simulink model "signal_processing_simulink_hw1"  (R2017b)
settings: Solver=FixedStepAuto  StartTime=0.0  StopTime=2  FixedStep=0.01  RelTol=1e-3
values from neighbouring files (symbols this model uses):
  f = fl(k)    [signal_processing_hw1.m]
  M2 = 5    [signal_processing_hw1.m]
libraries: commchan3 x1
settings Model: Creator=nlztrk  LastModifiedBy=anilo
settings CodeAppCC: StateflowObjectComments=on

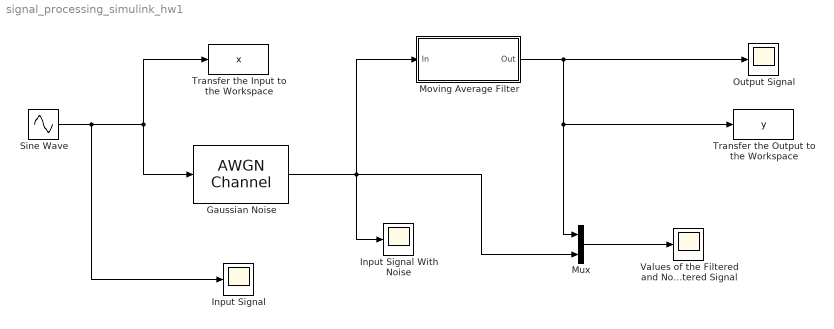
== system signal_processing_simulink_hw1 ==
  Gaussian Noise : commchan3/AWGN Channel  InputProcessing=Columns as channels (frame based)  seed=67  noiseMode=Variance from mask  EbNodB=10  EsNodB=10  SNRdB=10  bitsPerSym=1  Ps=1  Tsym=1  variance=0.2
  "Input Signal " : Scope
  Input Signal With Noise : Scope
  Moving Average Filter : Subsystem
  Mux : Mux  Inputs=2
  Output Signal : Scope
  Sine Wave : Sin  Amplitude=5  Frequency=2*pi*f  SampleTime=0.01
  Transfer the Input to the Workspace : ToWorkspace  VariableName=x  SampleTime=0.01
      settings: Save2DSignal=2-D array (concatenate along first dimension)
  "Transfer the Output to the Workspace " : ToWorkspace  VariableName=y  SampleTime=0.01
      settings: Save2DSignal=2-D array (concatenate along first dimension)
  "Values of the Filtered and Non-Filtered Signal " : Scope
  wires:
  Sine Wave/1 -> "Input Signal "/1, Gaussian Noise/1, Transfer the Input to the Workspace/1
  Moving Average Filter/1(Out) -> Mux/1, "Transfer the Output to the Workspace "/1, Output Signal/1
  Gaussian Noise/1 -> Mux/2, Input Signal With Noise/1, Moving Average Filter/1(In)
  Mux/1 -> "Values of the Filtered and Non-Filtered Signal "/1

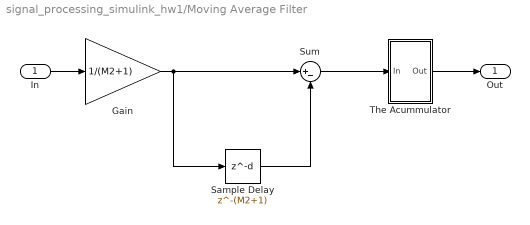
== system signal_processing_simulink_hw1/Moving Average Filter ==
  In : Inport
  Gain : Gain  Gain=1/(M2+1)
  Sample Delay : Delay  DelayLength=(M2+1)  InitialCondition=0  SampleTime=0.01
  Sum : Sum  Inputs=|+-
  The Acummulator : Subsystem
  Out : Outport
  wires:
  In/1 -> Gain/1
  Gain/1 -> Sample Delay/1, Sum/1
  Sample Delay/1 -> Sum/2
  Sum/1 -> The Acummulator/1(In)
  The Acummulator/1(Out) -> Out/1

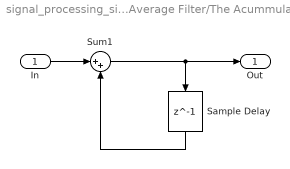
== system signal_processing_simulink_hw1/Moving Average Filter/The Acummulator ==
  In : Inport
  Sample Delay : Delay  DelayLength=1  InitialCondition=0  SampleTime=0.01
  Sum1 : Sum  Inputs=|++
  Out : Outport
  wires:
  In/1 -> Sum1/1
  Sum1/1 -> Out/1, Sample Delay/1
  Sample Delay/1 -> Sum1/2
